simulink model "task_1_2"  (R2023a)
settings: Solver=VariableStepAuto  StartTime=0.0  StopTime=3  RelTol=1e-3
model workspace (MAT data in the model file):
  f_s = 100000
libraries: commdigbbndpm3 x2, commfilt2 x2, commchan3 x1, commrandsrc3 x1, whdlio x1, dspsigops x1
settings Model: Creator=svdvl  LastModifiedBy=azamath
settings OptimizationCC: ReuseModelBlockBuffer=off

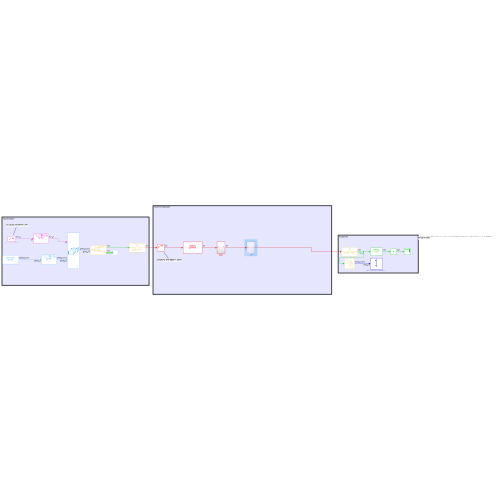
[thumbnail: Simulink's stored preview of the top-level diagram]
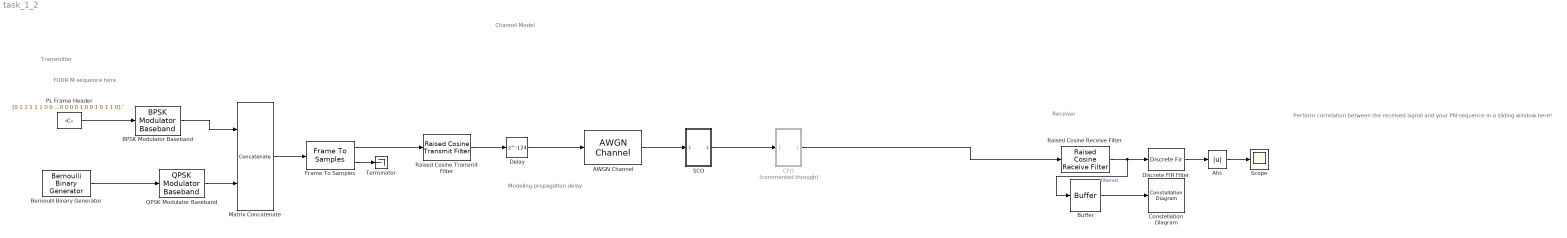
== system task_1_2 ==
  note: Modeling propagation delay
  note: Perform correlation between the received signal and your PN-sequence in a sliding window here!
  note: YOUR M-sequence here
  note: Receiver
  note: Transmitter
  note: Channel Model
  AWGN Channel : commchan3/AWGN Channel  LegacyMode=on  NoiseMethod="Signal to noise ratio  (SNR)"  noiseMode="Signal to noise ratio  (Es/No)"  EbNo=50  EsNo=500  SNR=10  BitsPerSymbol=2  SignalPower=1  SamplesPerSymbol=1  SymbolPeriod=1/f_s  VarianceSource=Parameter  Variance=1  RandomStream=Global stream  Seed=67  SimulateUsing=Code generation
  Abs : Abs  SaturateOnIntegerOverflow=off
  BPSK Modulator Baseband : commdigbbndpm3/BPSK Modulator Baseband  Ph=pi  outDtype=double  outWordLen=16  outUDDataType=sfix(16)  outFracLenMode=Best precision  outFracLen=15  outDataTypeStr=double  outLastDataTypeStr=double
      settings: LibrarySourceBlock=|
      | commhdldigbbndpm/BPSK
      | Modulator
      | Baseband
  Bernoulli Binary Generator : commrandsrc3/Bernoulli Binary Generator  ProbabilityOfZero=0.5  SeedSource=Auto  Seed=0  SampleTime=1/f_s  SamplesPerFrame=4096  OutputDataType=double  SimulateUsing=Interpreted execution
  Buffer : Buffer  N=1e3  OutputFrames=off
  CFO : Subsystem  Commented=through
  Constellation Diagram : ConstellationDiagram  WindowPosition=[443.000000,187.000000,600.000000,600.000000,]  ScopeFrameLocation=window  DefaultConfigurationName=comm.scopes.ConstellationDiagramBlockCfg
  Delay : Delay  DelayLength=124
  Discrete FIR Filter : DiscreteFir  Coefficients=fliplr([-1 1 1 1 1 1 -1 -1 -1 1 1 -1 1 1 1 -1 1 -1 1 -1 -1 -1 -1 1 -1 -1 1 -1 1 1 -1])
  Frame To Samples : whdlio/Frame To Samples  InterSampleIdleCycles=0  InterFrameIdleCycles=0  OutputSize=1  InterleaveSamples=off
  Matrix Concatenate : Concatenate  Mode=Multidimensional array
  PL Frame Header : Constant  Value=[0 1 1 1 1 1 0 0 0 1 1 0 1 1 1 0 1 0 1 0 0 0 0 1 0 0 1 0 1 1 0].'
  QPSK Modulator Baseband : commdigbbndpm3/QPSK Modulator Baseband  InType=Bit  Enc=Gray  Ph=pi/4  outDtype=double  outWordLen=16  outUDDataType=sfix(16)  outFracLenMode=Best precision  outFracLen=15  outDataTypeStr=double  outLastDataTypeStr=double
      settings: LibrarySourceBlock=|
      | commhdldigbbndpm/QPSK
      | Modulator
      | Baseband
  Raised Cosine Receive Filter : commfilt2/Raised Cosine Receive Filter  filtType=Square root  R=0.5  filtSpan=12  N=2  downFactor=2  downOffset=0  filterGain=1  RateOptions=Allow multirate processing  framing=Mute  checkCoeff=off  variableName=rcRxFilt  currentFiltSpan=10  D=5  inputOffset=0  sampMode=Mute  saveAsFlag=0  rateMode=Downsampling  checkGain=Normalized  launchFVT=on  roundingMode=Floor  overflowMode=off  coeffDataTypeStr=Inherit: Same word length as input  coeffMin=[]  coeffMax=[]  coeffLastDataTypeStr=Inherit: Same word length as input  accumDataTypeStr=Inherit: Same as product output  accumLastDataTypeStr=Inherit: Same as product output  outputDataTypeStr=Inherit: Same as accumulator  outputMin=[]  outputMax=[]  outputLastDataTypeStr=Inherit: Same as accumulator
  Raised Cosine Transmit Filter : commfilt2/Raised Cosine Transmit Filter  filtType=Square root  R=0.5  filtSpan=12  N=2  filterGain=1  RateOptions=Allow multirate processing  framing=Mute  checkCoeff=off  variableName=rcTxFilt1  checkGain=Normalized  sampMode=Mute  saveAsFlag=0  currentFiltSpan=10  D=5  launchFVT=on  roundingMode=Floor  overflowMode=off  coeffDataTypeStr=Inherit: Same word length as input  coeffMin=[]  coeffMax=[]  coeffLastDataTypeStr=Inherit: Same word length as input  outputDataTypeStr=Inherit: Same as accumulator  outputMin=[]  outputMax=[]  outputLastDataTypeStr=Inherit: Same as accumulator
  SCO : Subsystem
  Scope : Scope
  Terminator : Terminator
  wires:
  PL Frame Header/1 -> BPSK Modulator Baseband/1
  Frame To Samples/2 -> Terminator/1
  Matrix Concatenate/1 -> Frame To Samples/1
  Frame To Samples/1 -> Raised Cosine Transmit Filter/1
  QPSK Modulator Baseband/1 -> Matrix Concatenate/2
  Raised Cosine Transmit Filter/1 -> Delay/1
  Bernoulli Binary Generator/1 -> QPSK Modulator Baseband/1
  Raised Cosine Receive Filter/1 -> Buffer/1, Discrete FIR Filter/1  "filtered"
  Abs/1 -> Scope/1
  Discrete FIR Filter/1 -> Abs/1
  Buffer/1 -> Constellation Diagram/1
  BPSK Modulator Baseband/1 -> Matrix Concatenate/1
  CFO/1(Out1) -> Raised Cosine Receive Filter/1
  Delay/1 -> AWGN Channel/1
  AWGN Channel/1 -> SCO/1(In1)
  SCO/1(Out1) -> CFO/1(In1)

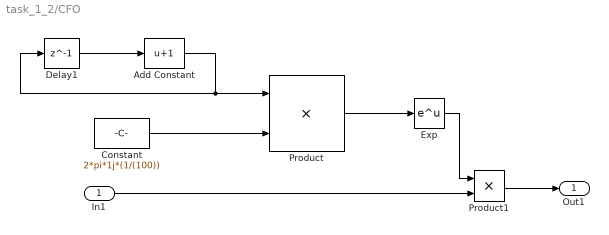
== system task_1_2/CFO ==
  In1 : Inport
  Add Constant : Bias  Bias=1  SaturateOnIntegerOverflow=off
  Constant : Constant  Value=2*pi*1j*(1/(100))
  Delay1 : Delay  DelayLength=1
  Exp : Math
  Product : Product
  Product1 : Product
  Out1 : Outport
  wires:
  In1/1 -> Product1/2
  Product1/1 -> Out1/1
  Delay1/1 -> Add Constant/1
  Exp/1 -> Product1/1
  Constant/1 -> Product/2
  Product/1 -> Exp/1
  Add Constant/1 -> Delay1/1, Product/1

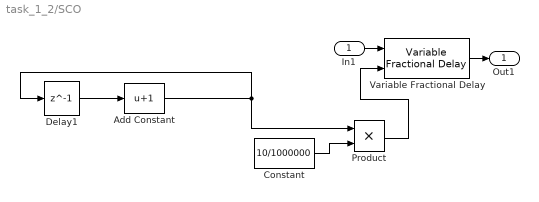
== system task_1_2/SCO ==
  In1 : Inport
  Add Constant : Bias  Bias=1  SaturateOnIntegerOverflow=off
  Constant : Constant  Value=10/1000000
  Delay1 : Delay  DelayLength=1
  Product : Product
  Variable Fractional Delay : dspsigops/Variable Fractional Delay  mode=OBSOLETE  modeActive=Linear  L=4  FarrowL=4  R=10  alpha=1  dmax=100  InputProcessing=Columns as channels (frame based)  ic=0  noDFT=off  fallbackFIR=Clip to the minimum value necessary for centered kernel  fallbackFarrow=Clip to the minimum value necessary for centered kernel  roundingMode=Zero  overflowMode=off
  Out1 : Outport
  wires:
  Variable Fractional Delay/1 -> Out1/1
  Constant/1 -> Product/2
  Product/1 -> Variable Fractional Delay/2
  In1/1 -> Variable Fractional Delay/1
  Add Constant/1 -> Product/1, Delay1/1
  Delay1/1 -> Add Constant/1
